simulink model "MotorControlLib"  (R2022b)
settings: Solver=FixedStepDiscrete  StartTime=0.0  StopTime=100  FixedStep=Ts  RelTol=1e-3  EnableMultiTasking=on
values from neighbouring files (symbols this model uses):
  BrkPoints : value not decoded    [MotorControl.sldd]
  CuttOffFreq_c = 4000.0    [MotorControl.sldd]
  d_q_Voltage_Limiter_max = 5.77    [MotorControl.sldd]
  dSoll = 0.0    [MotorControl.sldd]
  EMFobsLdGain = 50000.0    [MotorControl.sldd]
  EMFobsRS = 0.34    [MotorControl.sldd]
  Ki_dAxis = 180.0    [MotorControl.sldd]
  Ki_Iab_EMFobs = 0.0    [MotorControl.sldd]
  Ki_qAxis = 175.0    [MotorControl.sldd]
  Ki_Rpm = 10.0    [MotorControl.sldd]
  Kp_dAxis = 0.146    [MotorControl.sldd]
  Kp_Iab_EMFobs = 1.0    [MotorControl.sldd]
  Kp_qAxis = 0.146    [MotorControl.sldd]
  Kp_Rpm = 0.146    [MotorControl.sldd]
  MaxBckEMFVol_sat_neg = -12.0    [MotorControl.sldd]
  MaxBckEMFVol_sat_pos = 12.0    [MotorControl.sldd]
  Minus_1 = -1.0    [MotorControl.sldd]
  pwmTableData : value not decoded    [MotorControl.sldd]
  TqToIqConst = 1.0    [MotorControl.sldd]
  Ts = 5.0E-5    [MotorControl.sldd]
  TsIntern = 5.0E-5    [MotorControl.sldd]
undefined symbols (not defined in the file or in its folder): DiscIntNeverNeededParam, NumBits1, NumBits2, Slope1, Slope2
libraries: simulink x8, slpidlib x2, simulink_extras x2
(part 2 of 2)

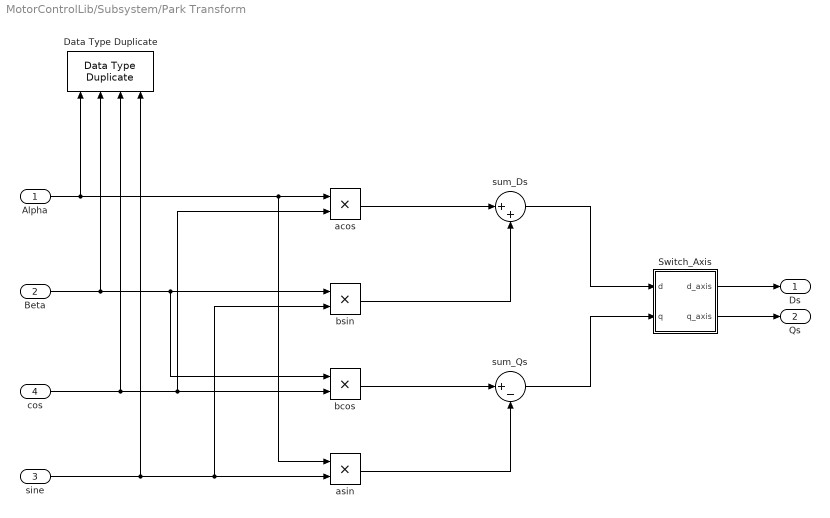
== system MotorControlLib/Subsystem/Park Transform ==
  Alpha : Inport
  Beta : Inport  Port=2
  sine : Inport  Port=3
  cos : Inport  Port=4
  Data Type Duplicate : DataTypeDuplicate  NumInputPorts=4
  Switch_Axis : Subsystem
  acos : Product  RndMeth=Simplest  OutDataTypeStr=Inherit: Same as first input
  asin : Product  RndMeth=Simplest  OutDataTypeStr=Inherit: Same as first input
  bcos : Product  OutDataTypeStr=Inherit: Inherit via back propagation  RndMeth=Simplest
  bsin : Product  OutDataTypeStr=Inherit: Inherit via back propagation  RndMeth=Simplest
  sum_Ds : Sum  Inputs=|++  RndMeth=Simplest  OutDataTypeStr=Inherit: Same as first input
  sum_Qs : Sum  Inputs=|+-  RndMeth=Simplest  OutDataTypeStr=Inherit: Same as first input
  Ds : Outport  VectorParamsAs1DForOutWhenUnconnected=off
  Qs : Outport  Port=2  VectorParamsAs1DForOutWhenUnconnected=off
  wires:
  Beta/1 -> Data Type Duplicate/2, bcos/1, bsin/1
  Switch_Axis/1(d_axis) -> Ds/1
  Switch_Axis/2(q_axis) -> Qs/1
  sum_Ds/1 -> Switch_Axis/1(d)
  sum_Qs/1 -> Switch_Axis/2(q)
  cos/1 -> Data Type Duplicate/3, bcos/2, acos/2
  asin/1 -> sum_Qs/2
  bcos/1 -> sum_Qs/1
  bsin/1 -> sum_Ds/2
  acos/1 -> sum_Ds/1
  Alpha/1 -> Data Type Duplicate/1, acos/1, asin/1
  sine/1 -> bsin/2, asin/2, Data Type Duplicate/4

== system MotorControlLib/CosSin/Sine-Cosine Lookup/Interpolation ==
  In1 : Inport
  In2 : Inport  Port=2
  Demux : Demux
  Product : Product  RndMeth=Simplest  OutDataTypeStr=Inherit: Same as first input
  Product1 : Product  RndMeth=Simplest  OutDataTypeStr=Inherit: Same as first input
  Sum3 : Sum  Inputs=|+-  RndMeth=Simplest  OutDataTypeStr=Inherit: Same as first input
  Sum4 : Sum  Inputs=|++  RndMeth=Simplest  OutDataTypeStr=Inherit: Same as first input
  Sum5 : Sum  Inputs=|+-  RndMeth=Simplest  OutDataTypeStr=Inherit: Same as first input
  Sum6 : Sum  Inputs=|++  RndMeth=Simplest  OutDataTypeStr=Inherit: Same as first input
  Out1 : Outport
  Out2 : Outport  Port=2
  wires:
  Sum4/1 -> Out1/1
  Sum6/1 -> Out2/1
  Demux/1 -> Sum3/1
  Sum5/1 -> Product1/1
  Demux/2 -> Sum3/2, Sum4/2
  In2/1 -> Product/2, Product1/2
  Product/1 -> Sum4/1
  Demux/4 -> Sum6/2, Sum5/2
  Product1/1 -> Sum6/1
  In1/1 -> Demux/1
  Sum3/1 -> Product/1
  Demux/3 -> Sum5/1

== system MotorControlLib/CosSin/Sine-Cosine Lookup/WrapUp ==
  In1 : Inport
  Compare To Zero : simulink/Logic and Bit Operations/Compare To Zero  relop=<  OutDataTypeStr=boolean
  Data Type Conversion : DataTypeConversion  OutDataTypeStr=uint16  ConvertRealWorld=Stored Integer (SI)  RndMeth=Simplest  SaturateOnIntegerOverflow=off
  If : If
  If Action Subsystem : Subsystem  TreatAsAtomicUnit=on
  If Action Subsystem1 : Subsystem  TreatAsAtomicUnit=on
  Merge : Merge
  convert_pu : Gain  Gain=1/(dlgSett.UpperSatLimit)  RndMeth=Simplest  OutDataTypeStr=Inherit: Same as input
  Out1 : Outport
  wires:
  In1/1 -> convert_pu/1
  If/1 -> If Action Subsystem/Action
  If/2 -> If Action Subsystem1/Action
  convert_pu/1 -> Compare To Zero/1, If Action Subsystem/1(In1), If Action Subsystem1/1(In1)
  If Action Subsystem/1(Out1) -> Merge/1
  If Action Subsystem1/1(Out1) -> Merge/2
  Compare To Zero/1 -> Data Type Conversion/1
  Data Type Conversion/1 -> If/1
  Merge/1 -> Out1/1

== system MotorControlLib/Position observer/EMF Observer Ia/DC Motor Model ==
  note: d/dt(i)
  note: Integrator
  Sig_Emfobs_PI_out : Inport
  In2 : Inport  Port=2
  In3 : Inport  Port=3
  Add5 : Sum  Inputs=-+--  OutDataTypeStr=Inherit: Same as first input
  Data Type Conversion : DataTypeConversion  SaturateOnIntegerOverflow=off  RndMeth=Floor
  Delay : Delay  DelayLength=1  InitialCondition=0  StateName=UnitDelayIntegratorPosObs
  Gain : Gain  Gain=TsIntern  ParamDataTypeStr=Inherit: Inherit from 'Gain'  OutMin=-100  OutMax=+100  OutDataTypeStr=single  SaturateOnIntegerOverflow=on
  Inductance : Gain  Gain=Ld  OutDataTypeStr=single
  Resistance : Gain  Gain=Rs  OutDataTypeStr=Inherit: Inherit via back propagation
  Sum : Sum  Inputs=|++  OutDataTypeStr=Inherit: Same as first input
  Unit Delay : UnitDelay  SampleTime=-1  HasFrameUpgradeWarning=on
  i_integrated_en8 : Outport
  wires:
  Unit Delay/1 -> Inductance/1
  Gain/1 -> Sum/1  "di_dt_times_Ts_En8"
  Sum/1 -> Delay/1, Data Type Conversion/1, Resistance/1  "i_integrated_en4"
  In2/1 -> Add5/2
  Resistance/1 -> Add5/1  "i_integrated_times_Rs_en8"
  Delay/1 -> Sum/2
  Sig_Emfobs_PI_out/1 -> Add5/3
  Add5/1 -> Unit Delay/1  "Va_all_16En4"
  Inductance/1 -> Gain/1  "di_dt_E9"
  Data Type Conversion/1 -> i_integrated_en8/1
  In3/1 -> Add5/4

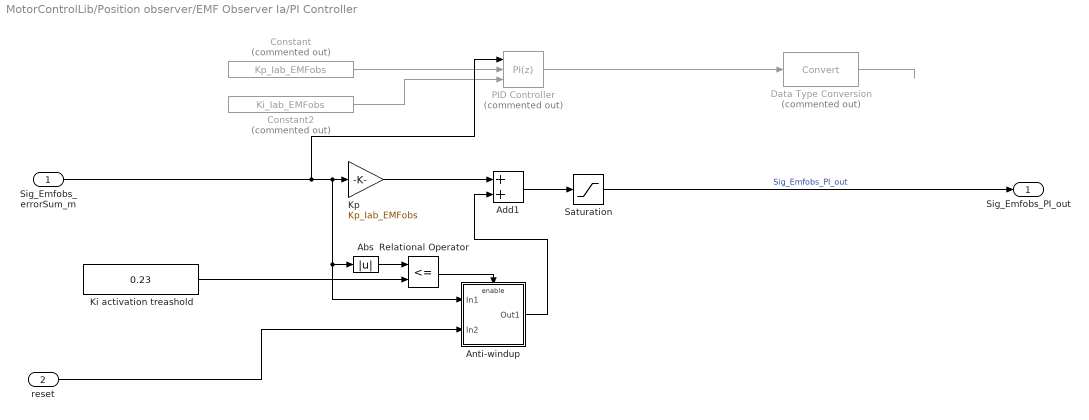
== system MotorControlLib/Position observer/EMF Observer Ia/PI Controller ==
  Sig_Emfobs_errorSum_m : Inport
  reset : Inport  Port=2
  Abs : Abs  SaturateOnIntegerOverflow=off
  Add1 : Sum
  Anti-windup : Subsystem
  Constant : Constant  Commented=on  Value=Kp_Iab_EMFobs
  Constant2 : Constant  Commented=on  Value=Ki_Iab_EMFobs
  Data Type Conversion : DataTypeConversion  Commented=on  SaturateOnIntegerOverflow=off  RndMeth=Floor
  Ki activation treashold : Constant  Value=0.23  OutDataTypeStr=single
  Kp : Gain  Gain=Kp_Iab_EMFobs  OutDataTypeStr=Inherit: Same as input
  PID Controller : slpidlib/PID Controller  Commented=on  Controller=PI  Form=Parallel  TimeDomain=Discrete-time  UseExternalTs=off  SampleTime=-1  IntegratorMethod=Forward Euler  FilterMethod=Forward Euler  ControllerParametersSource=external  P=1  I=1  UseKiTs=off  D=0  N=100  UseFilter=on  TunerSelectOption=Transfer Function Based (PID Tuner App)  ZeroCross=off  InitialConditionSource=internal  InitialConditionForIntegrator=0  InitialConditionForFilter=0  DifferentiatorICPrevScaledInput=0  ExternalReset=none  TrackingMode=off  Kt=1  LimitOutput=on  SatLimitsSource=internal  UpperSaturationLimit=MaxBckEMFVol_sat_pos  LowerSaturationLimit=MaxBckEMFVol_sat_neg  LinearizeAsGain=on  AntiWindupMode=clamping  Kb=1  LimitIntegrator=off  UpperIntegratorSaturationLimit=inf  LowerIntegratorSaturationLimit=-inf  POutMin=[]  POutMax=[]  IOutMin=[]  IOutMax=[]  DOutMin=[]  DOutMax=[]  NOutMin=[]  NOutMax=[]  SumOutMin=[]  SumOutMax=[]  SaturationOutMin=[]  SaturationOutMax=[]  PParamMin=[]  PParamMax=[]  IParamMin=[]  IParamMax=[]  DParamMin=[]  DParamMax=[]  NParamMin=[]  NParamMax=[]  KbParamMin=[]  KbParamMax=[]  KtParamMin=[]  KtParamMax=[]  KbOutMin=[]  KbOutMax=[]  KtOutMin=[]  KtOutMax=[]  IntegratorOutMin=[]  IntegratorOutMax=[]  FilterOutMin=[]  FilterOutMax=[]  SumI1OutMin=[]  SumI1OutMax=[]  SumI2OutMin=[]  SumI2OutMax=[]  SumI3OutMin=[]  SumI3OutMax=[]  SumI4OutMin=[]  SumI4OutMax=[]  SumDOutMin=[]  SumDOutMax=[]  DifferentiatorOutMin=[]  DifferentiatorOutMax=[]  FilterDiffOutCoefMin=[]  FilterDiffOutCoefMax=[]  ReciprocalOutMin=[]  ReciprocalOutMax=[]  SumDenOutMin=[]  SumDenOutMax=[]  SumNumOutMin=[]  SumNumOutMax=[]  DivideOutMin=[]  DivideOutMax=[]  UdiffTsProdOutMin=[]  UdiffTsProdOutMax=[]  NTsProdOutMin=[]  NTsProdOutMax=[]  UintegralTsProdOutMin=[]  UintegralTsProdOutMax=[]  UngainTsProdOutMin=[]  UngainTsProdOutMax=[]  ClampingZeroOutDataTypeStr=Inherit: Inherit via back propagation  ClampingZeroOutMin=[]  ClampingZeroOutMax=[]  FilterDenConstantOutDataTypeStr=Inherit: Inherit via back propagation  FilterDenConstantOutMin=[]  FilterDenConstantOutMax=[]  PCopyOutDataTypeStr=Inherit: Inherit via back propagation  PCopyOutMin=[]  PCopyOutMax=[]  NCopyOutDataTypeStr=Inherit: Inherit via back propagation  NCopyOutMin=[]  NCopyOutMax=[]  IntegratorContinuousStateAttributes=''  IntegratorStateMustResolveToSignalObject=off  IntegratorRTWStateStorageClass=Auto  FilterContinuousStateAttributes=''  FilterStateMustResolveToSignalObject=off  FilterRTWStateStorageClass=Auto  ParallelPVariant=ExternalParameters  IdealPVariant=Disabled  IVariant=ExternalParameters  DVariant=Disabled  IntegratorVariant=Discrete  SatVariant=Enabled  AWVariant=DiscClampingParallel  PCopyVariant=Disabled  TRVariant=Disabled  FdbkBlocksVariant=Forward  IdealPFdbkVariant=Disabled  SatFdbkVariant=Disabled  DerivativeFilterVariant=Disabled  NVariant=Disabled  NCopyVariant=Disabled_SignalSpec  FilterICVariant=Disabled  IntegratorICVariant=InternalICs  ExternalResetVariant=Disabled  TRSumVariant=Passthrough  SumFdbkVariant=Disabled  SumVariant=Sum_PI  TsampFilterVariant=InternalTs  TsampNgainVariant=Passthrough  TsampIntegralVariant=Passthrough  ExternalSaturationOutDataTypeStr=Inherit: Same as second input
  Relational Operator : RelationalOperator  Operator=<=  OutDataTypeStr=boolean  RndMeth=Simplest  InputSameDT=off
  Saturation : Saturate  UpperLimit=MaxBckEMFVol_sat_pos  LowerLimit=MaxBckEMFVol_sat_neg
  Sig_Emfobs_PI_out : Outport
  wires:
  PID Controller/1 -> Data Type Conversion/1
  Kp/1 -> Add1/1
  Anti-windup/1(Out1) -> Add1/2
  Ki activation treashold/1 -> Relational Operator/2
  Add1/1 -> Saturation/1
  Relational Operator/1 -> Anti-windup/Enable
  Constant/1 -> PID Controller/2
  Constant2/1 -> PID Controller/3
  Data Type Conversion/1 -> ?
  Sig_Emfobs_errorSum_m/1 -> PID Controller/1, Anti-windup/1(In1), Abs/1, Kp/1
  Saturation/1 -> Sig_Emfobs_PI_out/1  "Sig_Emfobs_PI_out"
  Abs/1 -> Relational Operator/1
  reset/1 -> Anti-windup/2(In2)

== system MotorControlLib/Position observer/EMF Observer Ia1/DC Motor Model ==
  note: Integrator
  note: d/dt(i)
  note: i
  In1 : Inport
  In2 : Inport  Port=2
  Add5 : Sum  Inputs=-+-  OutDataTypeStr=Inherit: Same as first input
  Delay : Delay  DelayLength=1  InitialCondition=0
  Gain : Gain  Gain=TsIntern  ParamDataTypeStr=Inherit: Inherit from 'Gain'  OutDataTypeStr=Inherit: Inherit via back propagation
  Inductance : Gain  Gain=Ld  OutDataTypeStr=Inherit: Same as input
  Resistance : Gain  Gain=Rs  OutDataTypeStr=Inherit: Inherit via back propagation
  Sum : Sum  Inputs=|++  OutDataTypeStr=Inherit: Same as first input
  Unit Delay : UnitDelay  SampleTime=-1  HasFrameUpgradeWarning=on
  Out1 : Outport
  wires:
  Gain/1 -> Sum/1
  Delay/1 -> Sum/2
  Inductance/1 -> Gain/1
  Sum/1 -> Resistance/1, Out1/1, Delay/1
  Resistance/1 -> Add5/1
  Unit Delay/1 -> Inductance/1
  In1/1 -> Add5/3
  Add5/1 -> Unit Delay/1
  In2/1 -> Add5/2

== system MotorControlLib/Position observer/EMF Observer Ia1/PI Controller ==
  In1 : Inport
  In2 : Inport  Port=2
  Add1 : Sum
  Add6 : Sum  Inputs=-+  InputSameDT=on
  Anti-windup : Subsystem
  Constant1 : Constant  Value=0.8  OutDataTypeStr=fixdt(1,32,2^-8,0)
  Kp : Gain  Gain=Kp_Iab_EMFobs  OutDataTypeStr=Inherit: Same as input
  Relational Operator : RelationalOperator  Operator=<=  OutDataTypeStr=boolean  RndMeth=Simplest  InputSameDT=off
  Saturation : Saturate  UpperLimit=MaxBckEMFVol_sat_pos  LowerLimit=MaxBckEMFVol_sat_neg
  Out1 : Outport
  wires:
  In2/1 -> Add6/2
  Add6/1 -> Anti-windup/1(In1), Relational Operator/1, Kp/1
  Anti-windup/1(Out1) -> Add1/2
  Constant1/1 -> Relational Operator/2
  In1/1 -> Add6/1
  Relational Operator/1 -> Anti-windup/Enable
  Add1/1 -> Saturation/1
  Kp/1 -> Add1/1
  Saturation/1 -> Out1/1

== system MotorControlLib/Position observer/EMF Observer Ia2/DC Motor Model ==
  note: Integrator
  note: d/dt(i)
  note: i
  Sig_Emfobs_PI_out : Inport
  In2 : Inport  Port=2
  Sig_Emfobs_PI_out1 : Inport  Port=3
  Add5 : Sum  Inputs=-+--  OutDataTypeStr=Inherit: Same as first input
  Delay : Delay  DelayLength=1  InitialCondition=0
  Gain : Gain  Gain=TsIntern  ParamDataTypeStr=Inherit: Inherit from 'Gain'  OutMin=-100  OutMax=+100  OutDataTypeStr=fixdt(1,16,2^-4,0)  SaturateOnIntegerOverflow=on
  Inductance : Gain  Gain=Ld  OutDataTypeStr=fixdt(1,16,2^9,0)
  Resistance : Gain  Gain=Rs  OutDataTypeStr=Inherit: Inherit via back propagation
  Sum : Sum  Inputs=|++  OutDataTypeStr=Inherit: Same as first input
  Unit Delay : UnitDelay  SampleTime=-1  HasFrameUpgradeWarning=on
  i_integrated_en8 : Outport
  wires:
  Sum/1 -> Resistance/1, i_integrated_en8/1, Delay/1
  Inductance/1 -> Gain/1
  Add5/1 -> Unit Delay/1
  Sig_Emfobs_PI_out/1 -> Add5/3
  Delay/1 -> Sum/2
  Resistance/1 -> Add5/1
  In2/1 -> Add5/2
  Gain/1 -> Sum/1
  Unit Delay/1 -> Inductance/1
  Sig_Emfobs_PI_out1/1 -> Add5/4

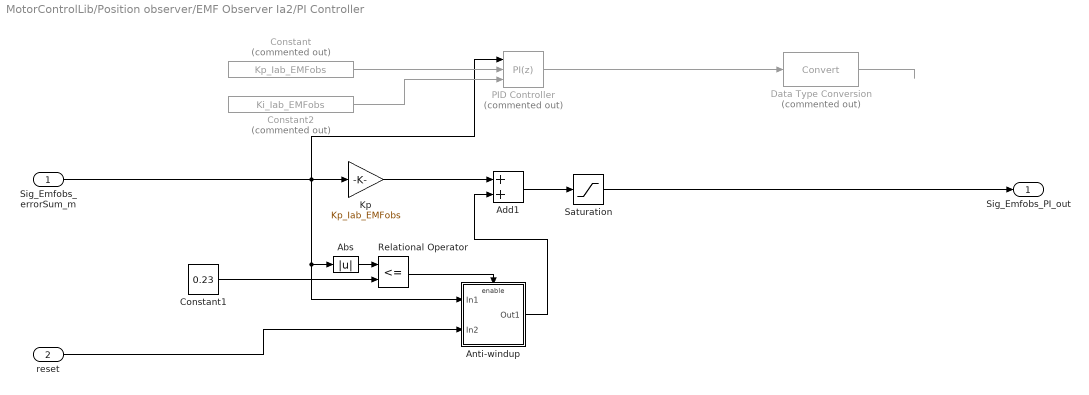
== system MotorControlLib/Position observer/EMF Observer Ia2/PI Controller ==
  Sig_Emfobs_errorSum_m : Inport
  reset : Inport  Port=2
  Abs : Abs  SaturateOnIntegerOverflow=off
  Add1 : Sum
  Anti-windup : Subsystem
  Constant : Constant  Commented=on  Value=Kp_Iab_EMFobs
  Constant1 : Constant  Value=0.23  OutDataTypeStr=fixdt(1,16,2^-8,0)
  Constant2 : Constant  Commented=on  Value=Ki_Iab_EMFobs
  Data Type Conversion : DataTypeConversion  Commented=on  SaturateOnIntegerOverflow=off  RndMeth=Floor
  Kp : Gain  Gain=Kp_Iab_EMFobs  ParamDataTypeStr=Inherit: Inherit from 'Gain'  OutDataTypeStr=Inherit: Same as input
  PID Controller : slpidlib/PID Controller  Commented=on  Controller=PI  Form=Parallel  TimeDomain=Discrete-time  UseExternalTs=off  SampleTime=-1  IntegratorMethod=Forward Euler  FilterMethod=Forward Euler  ControllerParametersSource=external  P=1  I=1  UseKiTs=off  D=0  N=100  UseFilter=on  TunerSelectOption=Transfer Function Based (PID Tuner App)  ZeroCross=off  InitialConditionSource=internal  InitialConditionForIntegrator=0  InitialConditionForFilter=0  DifferentiatorICPrevScaledInput=0  ExternalReset=none  TrackingMode=off  Kt=1  LimitOutput=on  SatLimitsSource=internal  UpperSaturationLimit=MaxBckEMFVol_sat_pos  LowerSaturationLimit=MaxBckEMFVol_sat_neg  LinearizeAsGain=on  AntiWindupMode=clamping  Kb=1  LimitIntegrator=off  UpperIntegratorSaturationLimit=inf  LowerIntegratorSaturationLimit=-inf  POutMin=[]  POutMax=[]  IOutMin=[]  IOutMax=[]  DOutMin=[]  DOutMax=[]  NOutMin=[]  NOutMax=[]  SumOutMin=[]  SumOutMax=[]  SaturationOutMin=[]  SaturationOutMax=[]  PParamMin=[]  PParamMax=[]  IParamMin=[]  IParamMax=[]  DParamMin=[]  DParamMax=[]  NParamMin=[]  NParamMax=[]  KbParamMin=[]  KbParamMax=[]  KtParamMin=[]  KtParamMax=[]  KbOutMin=[]  KbOutMax=[]  KtOutMin=[]  KtOutMax=[]  IntegratorOutMin=[]  IntegratorOutMax=[]  FilterOutMin=[]  FilterOutMax=[]  SumI1OutMin=[]  SumI1OutMax=[]  SumI2OutMin=[]  SumI2OutMax=[]  SumI3OutMin=[]  SumI3OutMax=[]  SumI4OutMin=[]  SumI4OutMax=[]  SumDOutMin=[]  SumDOutMax=[]  DifferentiatorOutMin=[]  DifferentiatorOutMax=[]  FilterDiffOutCoefMin=[]  FilterDiffOutCoefMax=[]  ReciprocalOutMin=[]  ReciprocalOutMax=[]  SumDenOutMin=[]  SumDenOutMax=[]  SumNumOutMin=[]  SumNumOutMax=[]  DivideOutMin=[]  DivideOutMax=[]  UdiffTsProdOutMin=[]  UdiffTsProdOutMax=[]  NTsProdOutMin=[]  NTsProdOutMax=[]  UintegralTsProdOutMin=[]  UintegralTsProdOutMax=[]  UngainTsProdOutMin=[]  UngainTsProdOutMax=[]  ClampingZeroOutDataTypeStr=Inherit: Inherit via back propagation  ClampingZeroOutMin=[]  ClampingZeroOutMax=[]  FilterDenConstantOutDataTypeStr=Inherit: Inherit via back propagation  FilterDenConstantOutMin=[]  FilterDenConstantOutMax=[]  PCopyOutDataTypeStr=Inherit: Inherit via back propagation  PCopyOutMin=[]  PCopyOutMax=[]  NCopyOutDataTypeStr=Inherit: Inherit via back propagation  NCopyOutMin=[]  NCopyOutMax=[]  IntegratorContinuousStateAttributes=''  IntegratorStateMustResolveToSignalObject=off  IntegratorRTWStateStorageClass=Auto  FilterContinuousStateAttributes=''  FilterStateMustResolveToSignalObject=off  FilterRTWStateStorageClass=Auto  ParallelPVariant=ExternalParameters  IdealPVariant=Disabled  IVariant=ExternalParameters  DVariant=Disabled  IntegratorVariant=Discrete  SatVariant=Enabled  AWVariant=DiscClampingParallel  PCopyVariant=Disabled  TRVariant=Disabled  FdbkBlocksVariant=Forward  IdealPFdbkVariant=Disabled  SatFdbkVariant=Disabled  DerivativeFilterVariant=Disabled  NVariant=Disabled  NCopyVariant=Disabled_SignalSpec  FilterICVariant=Disabled  IntegratorICVariant=InternalICs  ExternalResetVariant=Disabled  TRSumVariant=Passthrough  SumFdbkVariant=Disabled  SumVariant=Sum_PI  TsampFilterVariant=InternalTs  TsampNgainVariant=Passthrough  TsampIntegralVariant=Passthrough  ExternalSaturationOutDataTypeStr=Inherit: Same as second input
  Relational Operator : RelationalOperator  Operator=<=  OutDataTypeStr=boolean  RndMeth=Simplest  InputSameDT=off
  Saturation : Saturate  UpperLimit=MaxBckEMFVol_sat_pos  LowerLimit=MaxBckEMFVol_sat_neg
  Sig_Emfobs_PI_out : Outport
  wires:
  Saturation/1 -> Sig_Emfobs_PI_out/1
  Sig_Emfobs_errorSum_m/1 -> Kp/1, Anti-windup/1(In1), Abs/1, PID Controller/1
  Data Type Conversion/1 -> ?
  Constant2/1 -> PID Controller/3
  Constant/1 -> PID Controller/2
  Relational Operator/1 -> Anti-windup/Enable
  Add1/1 -> Saturation/1
  Constant1/1 -> Relational Operator/2
  Anti-windup/1(Out1) -> Add1/2
  Kp/1 -> Add1/1
  PID Controller/1 -> Data Type Conversion/1
  Abs/1 -> Relational Operator/1
  reset/1 -> Anti-windup/2(In2)

== system MotorControlLib/Start up/Logic after motor is stoped/Enabled Subsystem ==
  In1 : Inport
  Enable : EnablePort
  Detect Change : simulink/Logic and Bit Operations/Detect Change  vinit=0  OutDataTypeStr=boolean
  Out1 : Outport
  wires:
  Detect Change/1 -> Out1/1
  In1/1 -> Detect Change/1

== system MotorControlLib/Start up/Logic after motor is stoped/Enabled Subsystem1 ==
  Enable : EnablePort
  Add : Sum  OutDataTypeStr=uint16
  Constant : Constant  OutDataTypeStr=uint8
  Constant1 : Constant  Value=10000  OutDataTypeStr=uint16
  Relational Operator : RelationalOperator  Operator=<=  OutDataTypeStr=boolean  RndMeth=Simplest  InputSameDT=off
  Unit Delay1 : UnitDelay  SampleTime=-1  HasFrameUpgradeWarning=on
  Output : Outport
  wires:
  Add/1 -> Unit Delay1/1
  Unit Delay1/1 -> Relational Operator/1, Add/1
  Constant/1 -> Add/2
  Constant1/1 -> Relational Operator/2
  Relational Operator/1 -> Output/1

== system MotorControlLib/Subsystem/Park Transform/Switch_Axis ==
  d : Inport
  q : Inport  Port=2
  D_axis_aligned : Mux  Inputs=2
  Demux : Demux  Outputs=2
  Offset : Constant  Value=0  OutDataTypeStr=uint16  SampleTime=-1
  Q_axis_aligned : Mux  Inputs=2
  Switch : Switch  Criteria=u2 > Threshold  Threshold=1  RndMeth=Simplest  ZeroCross=off  SaturateOnIntegerOverflow=off  InputSameDT=off
  Unary_Minus : UnaryMinus
  d_axis : Outport  VectorParamsAs1DForOutWhenUnconnected=off
  q_axis : Outport  Port=2  VectorParamsAs1DForOutWhenUnconnected=off
  wires:
  D_axis_aligned/1 -> Switch/3
  Q_axis_aligned/1 -> Switch/1
  d/1 -> D_axis_aligned/1, Q_axis_aligned/2
  Offset/1 -> Switch/2
  Demux/1 -> d_axis/1
  Unary_Minus/1 -> Q_axis_aligned/1
  q/1 -> D_axis_aligned/2, Unary_Minus/1
  Switch/1 -> Demux/1
  Demux/2 -> q_axis/1

== system MotorControlLib/CosSin/Sine-Cosine Lookup/WrapUp/If Action Subsystem ==
  In1 : Inport
  Action Port : ActionPort  ActionPortLabel=if(u1 > 0)
  Convert_back : DataTypeConversion  RndMeth=Simplest  SaturateOnIntegerOverflow=off
  Convert_uint16 : DataTypeConversion  OutDataTypeStr=int16  SaturateOnIntegerOverflow=off  RndMeth=Floor
  Data Type Duplicate : DataTypeDuplicate
  Sum : Sum  Inputs=|+-  RndMeth=Simplest  OutDataTypeStr=Inherit: Same as first input
  Out1 : Outport
  wires:
  In1/1 -> Convert_uint16/1, Sum/1, Data Type Duplicate/1
  Convert_back/1 -> Data Type Duplicate/2, Sum/2
  Sum/1 -> Out1/1
  Convert_uint16/1 -> Convert_back/1

== system MotorControlLib/CosSin/Sine-Cosine Lookup/WrapUp/If Action Subsystem1 ==
  In1 : Inport
  Action Port : ActionPort  ActionPortLabel=else
  Convert_back : DataTypeConversion  RndMeth=Simplest  SaturateOnIntegerOverflow=off
  Convert_uint16 : DataTypeConversion  OutDataTypeStr=int16  RndMeth=Simplest  SaturateOnIntegerOverflow=off
  Data Type Duplicate : DataTypeDuplicate
  Sum : Sum  Inputs=|+-  RndMeth=Simplest  OutDataTypeStr=Inherit: Same as first input
  Out1 : Outport
  wires:
  Convert_uint16/1 -> Convert_back/1
  Convert_back/1 -> Data Type Duplicate/2, Sum/2
  In1/1 -> Convert_uint16/1, Sum/1, Data Type Duplicate/1
  Sum/1 -> Out1/1

== system MotorControlLib/Position observer/EMF Observer Ia/PI Controller/Anti-windup ==
  note: d/dt(i)
  note: Integrator
  In1 : Inport
  In2 : Inport  Port=2
  Enable : EnablePort
  Delay1 : Delay  DelayLength=1  InitialCondition=0  ExternalReset=Level
      settings: InputPortMap=u0,r5
  Gain1 : Gain  Gain=250e-6  ParamDataTypeStr=fixdt(1,16,2^-16,0)  OutDataTypeStr=single
  Ki : Gain  Gain=Ki_Iab_EMFobs  ParamDataTypeStr=Inherit: Inherit from 'Gain'  OutDataTypeStr=Inherit: Same as input
  Sum1 : Sum  Inputs=|++  OutDataTypeStr=fixdt(1,16,2^-8,0)
  Out1 : Outport
  wires:
  Sum1/1 -> Out1/1, Delay1/1
  Gain1/1 -> Sum1/1
  Delay1/1 -> Sum1/2
  In1/1 -> Ki/1
  Ki/1 -> Gain1/1
  In2/1 -> Delay1/2

== system MotorControlLib/Position observer/EMF Observer Ia1/PI Controller/Anti-windup ==
  note: Integrator
  note: d/dt(i)
  In1 : Inport
  Enable : EnablePort
  Delay1 : Delay  DelayLength=1  InitialCondition=0
  Gain1 : Gain  Gain=TsIntern  ParamDataTypeStr=Inherit: Inherit from 'Gain'  OutDataTypeStr=Inherit: Inherit via back propagation
  Ki : Gain  Gain=Ki_Iab_EMFobs  OutDataTypeStr=Inherit: Same as input
  Sum1 : Sum  Inputs=|++  OutDataTypeStr=Inherit: Same as first input
  Out1 : Outport
  wires:
  Ki/1 -> Gain1/1
  In1/1 -> Ki/1
  Delay1/1 -> Sum1/2
  Gain1/1 -> Sum1/1
  Sum1/1 -> Delay1/1, Out1/1

== system MotorControlLib/Position observer/EMF Observer Ia2/PI Controller/Anti-windup ==
  note: Integrator
  note: d/dt(i)
  In1 : Inport
  In2 : Inport  Port=2
  Enable : EnablePort
  Delay1 : Delay  DelayLength=1  InitialCondition=0  ExternalReset=Level
      settings: InputPortMap=u0,r5
  Gain1 : Gain  Gain=250e-6  ParamDataTypeStr=fixdt(1,16,2^-16,0)  OutDataTypeStr=fixdt(1,16,2^-12,0)
  Ki : Gain  Gain=Ki_Iab_EMFobs  ParamDataTypeStr=Inherit: Inherit from 'Gain'  OutDataTypeStr=Inherit: Same as input
      settings: AttributesFormatString=%<Gain>
  Sum1 : Sum  Inputs=|++  OutDataTypeStr=fixdt(1,16,2^-8,0)
  Out1 : Outport
  wires:
  Ki/1 -> Gain1/1
  In1/1 -> Ki/1
  Delay1/1 -> Sum1/2
  Gain1/1 -> Sum1/1
  Sum1/1 -> Delay1/1, Out1/1
  In2/1 -> Delay1/2
